simulink model "phy_model"  (R2021a)
settings: Solver=VariableStepAuto  StartTime=0.0  StopTime=inf  RelTol=1e-3
values from neighbouring files (symbols this model uses):
  Tb = 1/1200    (= 0.000833333333333)    [main.m]
  Ts = Tb / 128    (= 6.51041666667e-06)    [main.m]
libraries: commsink2 x1, commrandsrc3 x1, commchan3 x1, commfilt2 x1, dspsrcs4 x1
settings Model: Creator=fox  LastModifiedBy=fox

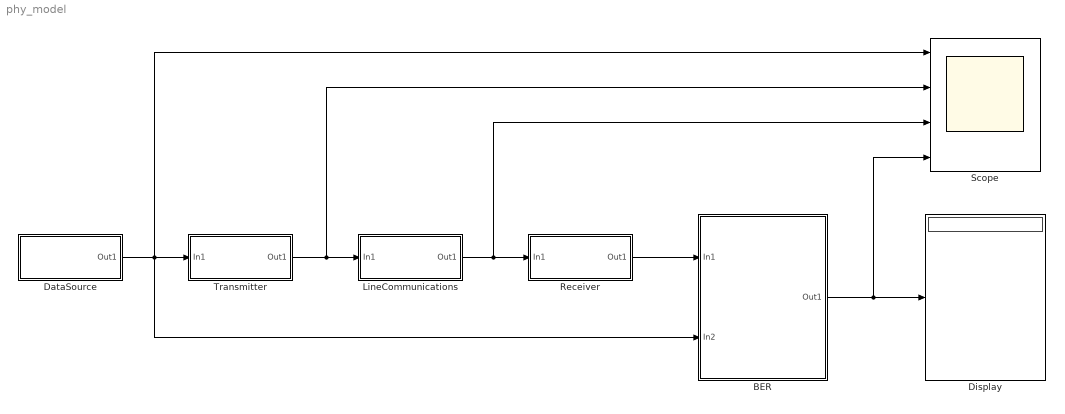
== system phy_model ==
  BER : Subsystem
  DataSource : Subsystem
  Display : Display
  LineCommunications : Subsystem
  Receiver : Subsystem
  Scope : Scope  NumInputPorts=4
  Transmitter : Subsystem
  wires:
  DataSource/1(Out1) -> BER/2(In2), Scope/1, Transmitter/1(In1)
  Transmitter/1(Out1) -> Scope/2, LineCommunications/1(In1)
  LineCommunications/1(Out1) -> Scope/3, Receiver/1(In1)
  Receiver/1(Out1) -> BER/1(In1)
  BER/1(Out1) -> Scope/4, Display/1

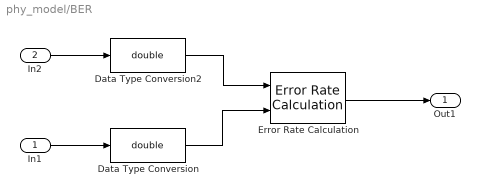
== system phy_model/BER ==
  In1 : Inport
  In2 : Inport  Port=2
  Data Type Conversion : DataTypeConversion  OutDataTypeStr=double
  Data Type Conversion2 : DataTypeConversion  OutDataTypeStr=double
  Error Rate Calculation : commsink2/Error Rate Calculation  N=1  st_delay=0  cp_mode=Entire frame  subframe=[]  PMode=Port  WsName=ErrorVec  RsMode2=off  stop=on  numErr=100  maxBits=1e8
  Out1 : Outport
  wires:
  In2/1 -> Data Type Conversion2/1
  In1/1 -> Data Type Conversion/1
  Error Rate Calculation/1 -> Out1/1
  Data Type Conversion2/1 -> Error Rate Calculation/1
  Data Type Conversion/1 -> Error Rate Calculation/2

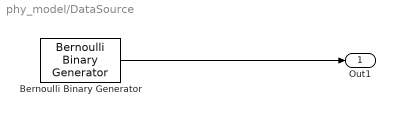
== system phy_model/DataSource ==
  Bernoulli Binary Generator : commrandsrc3/Bernoulli Binary Generator  ProbabilityOfZero=0.5  SeedSource=Auto  Seed=0  SampleTime=Tb  SamplesPerFrame=1  OutputDataType=boolean  SimulateUsing=Interpreted execution
  Out1 : Outport
  wires:
  Bernoulli Binary Generator/1 -> Out1/1

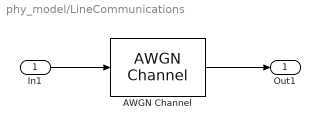
== system phy_model/LineCommunications ==
  In1 : Inport
  AWGN Channel : commchan3/AWGN Channel  InputProcessing=Columns as channels (frame based)  seed=67  noiseMode="Signal to noise ratio  (Eb/No)"  EbNodB=0  EsNodB=10  SNRdB=10  bitsPerSym=1  Ps=0.5  Tsym=Tb  variance=1
  Out1 : Outport
  wires:
  In1/1 -> AWGN Channel/1
  AWGN Channel/1 -> Out1/1

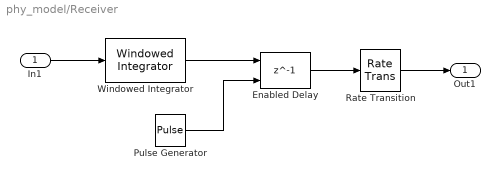
== system phy_model/Receiver ==
  In1 : Inport
  Enabled Delay : Delay  DelayLength=1  ShowEnablePort=on
      settings: InputPortMap=u0,e6
  Pulse Generator : DiscretePulseGenerator  Period=Tb/Ts  PhaseDelay=Tb/Ts-1  SampleTime=Ts
  Rate Transition : RateTransition  Integrity=off  OutPortSampleTime=Tb
  Windowed Integrator : commfilt2/Windowed Integrator  integperiod=Tb/Ts  InputProcessing=Columns as channels (frame based)  roundingMode=Floor  overflowMode=off  coeffDataTypeStr=Inherit: Same word length as input  coeffMin=[]  coeffMax=[]  coeffLastDataTypeStr=Inherit: Same word length as input  accumDataTypeStr=Inherit: Same as product output  accumLastDataTypeStr=Inherit: Same as product output  outputDataTypeStr=Inherit: Same as accumulator  outputMin=[]  outputMax=[]  outputLastDataTypeStr=Inherit: Same as accumulator
      settings: SourceProductBaseCode=CM
  Out1 : Outport
  wires:
  In1/1 -> Windowed Integrator/1
  Windowed Integrator/1 -> Enabled Delay/1
  Pulse Generator/1 -> Enabled Delay/2
  Rate Transition/1 -> Out1/1
  Enabled Delay/1 -> Rate Transition/1

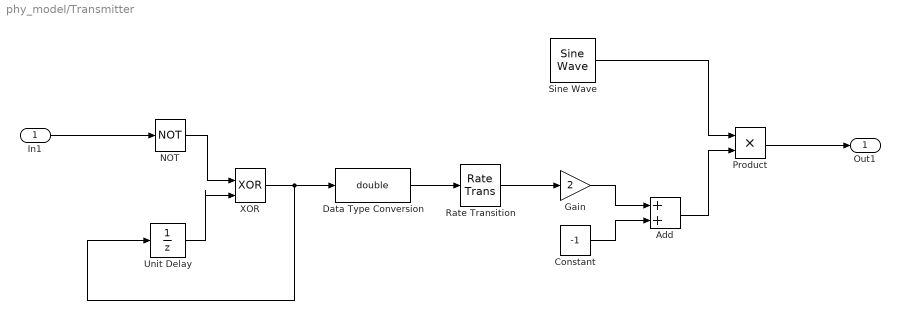
== system phy_model/Transmitter ==
  In1 : Inport
  Add : Sum
  Constant : Constant  Value=-1
  Data Type Conversion : DataTypeConversion  OutDataTypeStr=double
  Gain : Gain  Gain=2
  NOT : Logic  Operator=NOT  IconShape=distinctive  AllPortsSameDT=off  OutDataTypeStr=boolean
  Product : Product
  Rate Transition : RateTransition  Integrity=off  Deterministic=off  OutPortSampleTime=Ts
  Sine Wave : dspsrcs4/Sine Wave  Amplitude=1  Frequency=1800  Phase=0  SampleMode=Discrete  OutComplex=Real  CompMethod=Trigonometric fcn  TableSize=Speed  SampleTime=Ts  SamplesPerFrame=1  ResetState=Restart at time zero  OutputFrames=off  dataType=double  wordLen=16  udDataType=sfix(16)  fracBitsMode=Best precision  numFracBits=15  OutDataTypeStr=double  LastOutDataTypeStr=double
  Unit Delay : UnitDelay  SampleTime=-1  HasFrameUpgradeWarning=on
  XOR : Logic  Operator=XOR  IconShape=distinctive  AllPortsSameDT=off  OutDataTypeStr=boolean
  Out1 : Outport
  wires:
  Product/1 -> Out1/1
  Data Type Conversion/1 -> Rate Transition/1
  NOT/1 -> XOR/1
  XOR/1 -> Unit Delay/1, Data Type Conversion/1
  Gain/1 -> Add/1
  Constant/1 -> Add/2
  Add/1 -> Product/2
  Sine Wave/1 -> Product/1
  In1/1 -> NOT/1
  Rate Transition/1 -> Gain/1
  Unit Delay/1 -> XOR/2
